simulink model "ContainerVessel"  (Simulink 6.3)
settings: Solver=ode3  StartTime=0.0  StopTime=600.0  FixedStep=0.1  RelTol=1e-3
libraries: simulink x2
settings Model: LastModifiedBy=Hung Nguyen

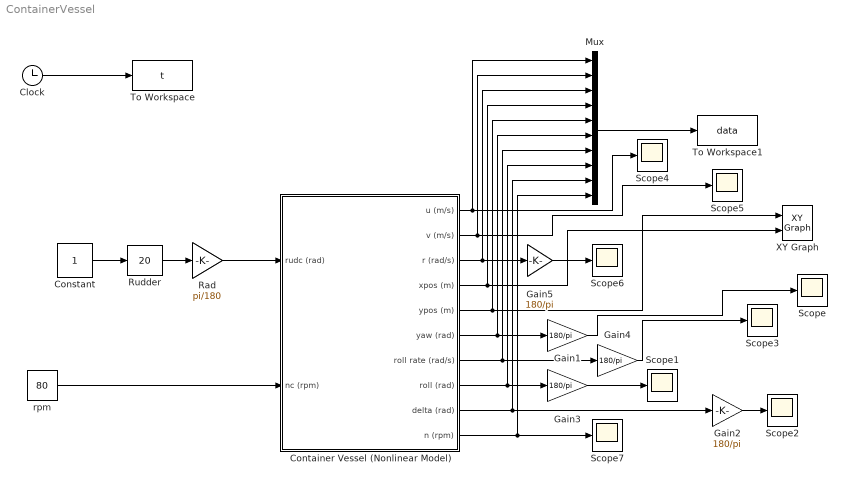
== system ContainerVessel ==
  Clock : Clock
      settings: Decimation=10
  Constant : Constant
  Container Vessel (Nonlinear Model) : Subsystem
  Gain{1..5} (5 alike) : Gain  Gain=180/pi
  Mux : Mux  Inputs=10
  Rad : Gain  Gain=pi/180  SaturateOnIntegerOverflow=on
  Rudder : simulink/Math Operations/Slider Gain  low=0  gain=20  high=360
  Scope{,1..7} (8 alike) : Scope
      Scope1 settings: YMin=-9  YMax=1
      Scope2 settings: SaveName=ScopeData2
      Scope3 settings: SaveName=ScopeData3
      Scope4 settings: YMin=-9  YMax=1  SaveName=ScopeData4
      Scope5 settings: YMin=-9  YMax=1  SaveName=ScopeData5
      Scope6 settings: YMin=-9  YMax=1  SaveName=ScopeData6
      Scope7 settings: SaveName=ScopeData7
  To Workspace : ToWorkspace  VariableName=t  SampleTime=-1  SaveFormat=Array
  To Workspace1 : ToWorkspace  VariableName=data  SampleTime=-1  SaveFormat=Array
      settings: Decimation=2
  XY Graph : simulink/Sinks/XY Graph  xmin=-1000  xmax=2000  ymin=-1000  ymax=2000  st=-1
  rpm : Constant  Value=80
  wires:
  Clock/1 -> To Workspace/1
  rpm/1 -> Container Vessel (Nonlinear Model)/2(nc (rpm))
  Container Vessel (Nonlinear Model)/4(xpos (m)) -> XY Graph/2, Mux/4
  Container Vessel (Nonlinear Model)/5(ypos (m)) -> XY Graph/1, Mux/5
  Container Vessel (Nonlinear Model)/6(yaw (rad)) -> Gain1/1, Mux/6
  Gain1/1 -> Scope/1
  Container Vessel (Nonlinear Model)/9(delta (rad)) -> Gain2/1, Mux/9
  Gain2/1 -> Scope2/1
  Container Vessel (Nonlinear Model)/8(roll (rad)) -> Gain3/1, Mux/8
  Gain3/1 -> Scope1/1
  Container Vessel (Nonlinear Model)/7(roll rate (rad/s)) -> Gain4/1, Mux/7
  Gain4/1 -> Scope3/1
  Mux/1 -> To Workspace1/1
  Container Vessel (Nonlinear Model)/1(u (m/s)) -> Scope4/1, Mux/1
  Container Vessel (Nonlinear Model)/2(v (m/s)) -> Scope5/1, Mux/2
  Container Vessel (Nonlinear Model)/3(r (rad/s)) -> Gain5/1, Mux/3
  Gain5/1 -> Scope6/1
  Container Vessel (Nonlinear Model)/10(n (rpm)) -> Scope7/1, Mux/10
  Constant/1 -> Rudder/1
  Rudder/1 -> Rad/1
  Rad/1 -> Container Vessel (Nonlinear Model)/1(rudc (rad))

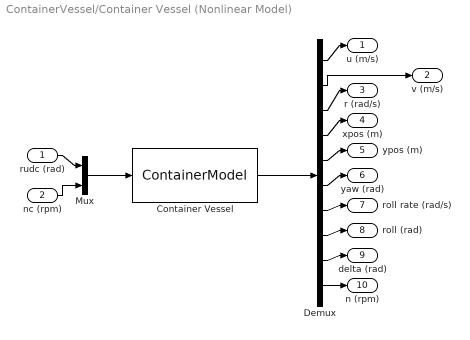
== system ContainerVessel/Container Vessel (Nonlinear Model) ==
  rudc (rad) : Inport
  nc (rpm) : Inport  Port=2
  Container Vessel : S-Function  FunctionName=ContainerModel
  Demux : Demux  Outputs=10
  Mux : Mux  Inputs=2
  u (m/s) : Outport
  v (m/s) : Outport  Port=2
  r (rad/s) : Outport  Port=3
  xpos (m) : Outport  Port=4
  ypos (m) : Outport  Port=5
  yaw (rad) : Outport  Port=6
  roll rate (rad/s) : Outport  Port=7
  roll (rad) : Outport  Port=8
  delta (rad) : Outport  Port=9
  n (rpm) : Outport  Port=10
  wires:
  Mux/1 -> Container Vessel/1
  Container Vessel/1 -> Demux/1
  Demux/1 -> u (m/s)/1
  Demux/2 -> v (m/s)/1
  Demux/3 -> r (rad/s)/1
  Demux/4 -> xpos (m)/1
  Demux/5 -> ypos (m)/1
  rudc (rad)/1 -> Mux/1
  Demux/6 -> yaw (rad)/1
  nc (rpm)/1 -> Mux/2
  Demux/7 -> roll rate (rad/s)/1
  Demux/8 -> roll (rad)/1
  Demux/9 -> delta (rad)/1
  Demux/10 -> n (rpm)/1
